simulink model "power_BoostConverter_feedback"  (R2017b)
settings: Solver=VariableStepAuto  StartTime=0.0  StopTime=0.01  MaxStep=1e-4  RelTol=1e-4  EnableMultiTasking=on
values from neighbouring files (symbols this model uses):
  C = 1e-6    (= 1e-06)    [audiotest.m]    (also in bridge.m; sallenkey.m = 1e-08)
  L = 4*C    (= 4e-06)    [audiotest.m]    (also in bridge.m = 6.4e-05)
  R = 8    [audiotest.m]    (also in bridge.m = 4; sallenkey.m = 2000)
  Rc = 1000    [audiotest.m]
  Ts = 1/Fs    (= 2.26757369615e-06)    [audiotest.m]
libraries: powerlib x12, powerlib_meascontrol x2, peGeneralControl x1
Description:
  | Copyright 2008-2017 The MathWorks, Inc.
settings Model: SimulationMode=rapid-accelerator  Creator=MathWorks  LastModifiedBy=s1246836
settings SolverCC: SolverResetMethod=Robust  DecoupledContinuousIntegration=on
settings DataIOCC: ReturnWorkspaceOutputs=on
settings OptimizationCC: EfficientFloat2IntCast=on  LifeSpan=inf
settings DebuggingCC: ReadBeforeWriteMsg=DisableAll  WriteAfterWriteMsg=DisableAll  WriteAfterReadMsg=DisableAll  UnconnectedInputMsg=none  UnconnectedOutputMsg=none  UnconnectedLineMsg=none  UniqueDataStoreMsg=error  StrictBusMsg=ErrorOnBusTreatedAsVector  SFUnexpectedBacktrackingDiag=warning  SFNoUnconditionalDefaultTransitionDiag=warning  SFExecutionAtInitializationDiag=none
settings ModelReferenceCC: UpdateModelReferenceTargets=IfOutOfDate
settings SFSimCC: SFSimEcho=off
settings CodeAppCC: StateflowObjectComments=on
settings GRTTargetCC: TargetLangStandard=C89/C90 (ANSI)  GeneratePreprocessorConditionals=Disable all
settings ConfigComp: CovMetricSettings=dw  CovHtmlReporting=on  CovSaveCumulativeToWorkspaceVar=on  CovSaveSingleToWorkspaceVar=on  CovExternalEMLEnable=off
settings SimscapeCC: SimscapeNormalizeSystem=off

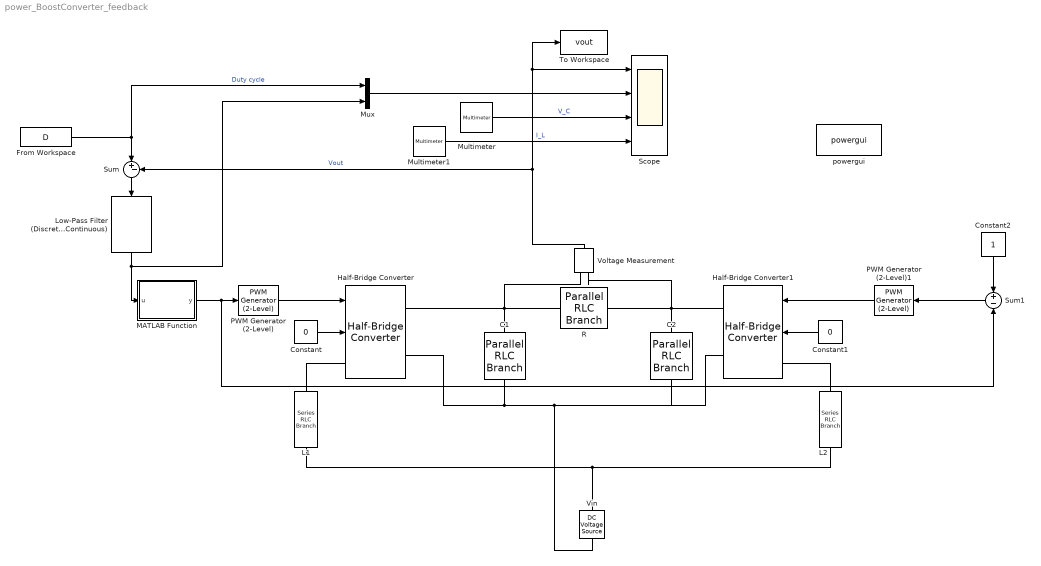
== system power_BoostConverter_feedback ==
  C1 : powerlib/Elements/Parallel RLC Branch  LConnTagsString=a  RConnTagsString=__new0  BranchType=RC  Resistance=Rc  Inductance=1e-3  SetiL0=off  InitialCurrent=0  Capacitance=C  Setx0=on  InitialVoltage=7.4  Measurements=Branch voltage
  C2 : powerlib/Elements/Parallel RLC Branch  LConnTagsString=a  RConnTagsString=__new0  BranchType=RC  Resistance=Rc  Inductance=1e-3  SetiL0=off  InitialCurrent=0  Capacitance=C  Setx0=on  InitialVoltage=7.4  Measurements=Branch voltage
  Constant : Constant  Value=0
  Constant1 : Constant  Value=0
  Constant2 : Constant
  From Workspace : FromWorkspace  VariableName=D  SampleTime=Ts
  Half-Bridge Converter : powerlib/Power Electronics/Half-Bridge Converter  ModelType=Switching devices  Ron=1e-3  Rs=1e6  Cs=inf  Vforward=[0,0]  Ron_Diode=1e-3  Rs_Diode=1e6  Cs_Diode=inf  Vf_Diode=1e-3  Rs_CurrentSource=inf
      settings: SourceProductName=Simscape Power Systems  SourceProductBaseCode=PS
  Half-Bridge Converter1 : powerlib/Power Electronics/Half-Bridge Converter  ModelType=Switching devices  Ron=1e-3  Rs=1e6  Cs=inf  Vforward=[0,0]  Ron_Diode=1e-3  Rs_Diode=1e6  Cs_Diode=inf  Vf_Diode=1e-3  Rs_CurrentSource=inf
      settings: SourceProductName=Simscape Power Systems  SourceProductBaseCode=PS
  L1 : powerlib/Elements/Series RLC Branch  LConnTagsString=__new0  RConnTagsString=__new0  BranchType=L  Resistance=1e-3  Inductance=L  SetiL0=off  InitialCurrent=0  Capacitance=1e-6  Setx0=off  InitialVoltage=0  Measurements=Branch current
  L2 : powerlib/Elements/Series RLC Branch  LConnTagsString=__new0  RConnTagsString=__new0  BranchType=L  Resistance=1e-3  Inductance=L  SetiL0=off  InitialCurrent=0  Capacitance=1e-6  Setx0=off  InitialVoltage=0  Measurements=Branch current
  Low-Pass Filter (Discrete or Continuous) : peGeneralControl/Low-Pass Filter (Discrete or Continuous)  K=1  T=1/20e3  B=inf  A=-inf  Ts=Ts
  MATLAB Function : MATLAB Function  TreatAsAtomicUnit=on
  Multimeter : powerlib/Measurements/Multimeter  PhasorSimulation=off  OutputType=Complex  sel=[1 2]  L=6  Gain=[1 1]  yselected={'Ub: C1','Ub: C2'};  PSBOutputType=1  PSBequivalent=0  AxesSetting=[0,0.1,-100,100]  Display=0  SavedBlockNames=-11
  Multimeter1 : powerlib/Measurements/Multimeter  PhasorSimulation=off  OutputType=Complex  sel=[4 5]  L=6  Gain=[1 1]  yselected={'Ib: L1','Ib: L2'};  PSBOutputType=1  PSBequivalent=0  AxesSetting=[0,0.1,-100,100]  Display=0  SavedBlockNames=-11
  Mux : Mux  Inputs=2
  PWM Generator (2-Level) : powerlib_meascontrol/Pulse & Signal Generators/PWM Generator (2-Level)  ModulatorType=Single-phase half-bridge (2 pulses)  ModulatorMode=Unsynchronized  Fc=1e6  Pc=90  nF=27  MinMax="[ 0  1 ]"  SamplingTechnique=Natural  ModulatingSignals=off  m=0.8  Freq=60  Phase=0  Ts=0  ShowCarrierOutport=off
      settings: SourceProductName=Simscape Power Systems
  PWM Generator (2-Level)1 : powerlib_meascontrol/Pulse & Signal Generators/PWM Generator (2-Level)  ModulatorType=Single-phase half-bridge (2 pulses)  ModulatorMode=Unsynchronized  Fc=1e6  Pc=90  nF=27  MinMax="[ 0  1 ]"  SamplingTechnique=Natural  ModulatingSignals=off  m=0.8  Freq=60  Phase=0  Ts=0  ShowCarrierOutport=off
      settings: SourceProductName=Simscape Power Systems
  R : powerlib/Elements/Parallel RLC Branch  LConnTagsString=a  RConnTagsString=__new0  BranchType=R  Resistance=R  Inductance=1e-3  SetiL0=off  InitialCurrent=0  Capacitance=C  Setx0=off  InitialVoltage=0  Measurements=Branch voltage and current
  Scope : Scope  NumInputPorts=4
  Sum : Sum  Inputs=|+-
  Sum1 : Sum  Inputs=+-
  To Workspace : ToWorkspace  VariableName=vout  SampleTime=Ts
  Vin : powerlib/Electrical Sources/DC Voltage Source  Amplitude=3.7  Measurements=None
  Voltage Measurement : powerlib/Measurements/Voltage Measurement  PhasorSimulation=off  OutputType=Complex  PSBequivalent=0
  powergui : powerlib/powergui  Priority=1  SimulationMode=Continuous  SampleTime=50e-6  frequency=60  Iterations=50  frequencyindice=0  Pbase=100e6  ErrMax=1e-4  UnitsV=kV  UnitsW=MW  buscounter=0  FunctionMessages=off  echomessages=off  EnableUseOfTLC=off  CurrentSourceSwitches=off  DisableSnubberDevices=off  DisableRonSwitches=off  DisableVfSwitches=off  DisplayEquations=off  SolverType=Tustin/Backward Euler (TBE)  Interpol=off  ExternalGateDelay=off  methode=off  Ts=100  x0status=blocks  SPID=on  SwTol=0  HookPort=off  RestoreLinks=warning  ResistiveCurrentMeasurement=off  Frange=[0:2:500]  Ylog=off  Xlog=on  ShowGrid=off  save=off  variable=ZData  structure=0  ZoomFFT=off  StartTime=0.0  cycles=1  DisplayStyle=1  fundamental=60  FreqAxis=off  MaxFrequency=1000  frequencyindicesteady=1  RmsSteady=1  display=off
  wires:
  Voltage Measurement/1 -> Sum/2, To Workspace/1, Scope/1  "Vout"
  Multimeter/1 -> Scope/3  "V_C"
  Constant/1 -> Half-Bridge Converter/2
  Constant1/1 -> Half-Bridge Converter1/2
  MATLAB Function/1(y) -> Sum1/2, PWM Generator (2-Level)/1
  From Workspace/1 -> Sum/1, Mux/1  "Duty cycle"
  Multimeter1/1 -> Scope/4  "I_L"
  Sum1/1 -> PWM Generator (2-Level)1/1
  Mux/1 -> Scope/2
  Sum/1 -> Low-Pass Filter (Discrete or Continuous)/1
  Constant2/1 -> Sum1/1
  PWM Generator (2-Level)/1 -> Half-Bridge Converter/1
  PWM Generator (2-Level)1/1 -> Half-Bridge Converter1/1
  Low-Pass Filter (Discrete or Continuous)/1 -> Mux/2, MATLAB Function/1(u)
  connections:
  Half-Bridge Converter1/RConn2 -- C2/RConn1 -- Vin/LConn1 -- Half-Bridge Converter/RConn2 -- C1/RConn1
  Voltage Measurement/LConn1 -- Half-Bridge Converter/RConn1 -- R/LConn1 -- C1/LConn1
  L1/LConn1 -- Vin/RConn1 -- L2/LConn1
  Half-Bridge Converter/LConn1 -- L1/RConn1
  Half-Bridge Converter1/LConn1 -- L2/RConn1
  R/RConn1 -- Half-Bridge Converter1/RConn1 -- Voltage Measurement/LConn2 -- C2/LConn1

== matlab function power_BoostConverter_feedback/MATLAB Function ==
  data: u input; y output
function y = fcn(u)
y=2./(u+2+sqrt(4+u.^2));
%y=yp*2-1
